simulink model "EPT"  (R2019b)
settings: Solver=FixedStepDiscrete  StartTime=0.0  StopTime=5  FixedStep=0.005  RelTol=1e-3  EnableMultiTasking=on
PreLoadFcn:
  | try, model_open; catch, disp('Error occurred while executing model pre-load callback: model_open.m'); disp('Please assure that the MATLAB working directory is set to the model directory before opening.'); end
InitFcn:
  | try, model_open; catch, end
undefined symbols (not defined in the file or in its folder): Bridge, GCM, H, ln, raptor_get_param_eval, raptor_get_safe_string, raptor_xcp_function
libraries: Raptor_lib x2810, simulink x374, hdlsllib x19
(part 16 of 45)

== system EPT/Foreground_TimeBase_5ms/CAN/CAN2_exec/BCU vs ITRI//ARTC/Remote DAG2-5EA ==
  Enable : EnablePort
  Trigger : TriggerPort  VariantControl=Variant  PortDimensions=1
  Data Type Conversion{1..8} (8 alike) : DataTypeConversion
  Fcn{1..8} (8 alike) : Fcn  Expr=(u(1)+40)/0.5
  raptor_can_txmsg : Raptor_lib/CAN/raptor_can_txmsg  canDefinition=struct('dbcFile', 'BCUvsRMDA_CMU.dbc','message', 'RemoteDAG_5EA','comment', '','signals', {{'CMU2_Tcell_T01','CMU2_Tcell_T02','CMU2_Tcell_T03','CMU2_Tcell_T04','CMU2_Tcell_T05','CMU2_Tcell_T06','CMU2_Tcell_T07','CMU2_Tcell_T08'}},'enabled', [ 1 1 1 1 1 1 1 1;],'canBus', '''CAN2''','messageID', [ 1514;],'idMask', [ 536870911;],'payloadMask', [],'payloadValue', [],'period', [ 0;],'mailbox', '','queueSize', [ 1;],'label', [ 0;],'ver', [ 2;],'showID', [ 0;],'showRaw', [ 0;],'fill', [ 0;],'editID', [ 0;],'signalOrder', [ 1;])  canBus='CAN2'  queueSize=1  payloadMask=[]  payloadValue=[]  period=0  showID=0  label=0  idMask=hex2dec('1FFFFFFF')  fill=0  id=1514  showRaw=0  signalOrder=1  signalInfo={{struct('Name', 'CMU2_Tcell_T01','Startbit', [ 0;],'SignalSize', [ 8;],'ByteOrder', 'BigEndian','ValueType', 'UNSIGNED','Class', 'uint8','Signed', [ 0;],'Factor', [ 1;],'Offset', [ 0;],'Min', [ 0;],'Max', [ 0;],'Units', '','Comment', '','StartBit', [ 0;]),struct('Name', 'CMU2_Tcell_T02','Startbit', [ 0;],'SignalSize', [ 8;],'ByteOrder', 'BigEndian','ValueType', 'UNSIGNED','Class', 'uint8','Signed', [ 0;],'Factor', [ 1;],'Offset', [ 0;],'Min', [ 0;],'Max', [ 0;],'Units', '','Comment', '','StartBit', [ 8;]),struct('Name', 'CMU2_Tcell_T03','Startbit', [ 0;],'SignalSize', [ 8;],'ByteOrder', 'BigEndian','ValueType', 'UNSIGNED','Class', 'uint8','Signed', [ 0;],'Factor', [ 1;],'Offset', [ 0;],'Min', [ 0;],'Max', [ 0;],'Units', '','Comment', '','StartBit', [ 16;]),struct('Name', 'CMU2_Tcell_T04','Startbit', [ 0;],'SignalSize', [ 8;],'ByteOrder', 'BigEndian','ValueType', 'UNSIGNED','Class', 'uint8','Signed', [ 0;],'Factor', [ 1;],'Offset', [ 0;],'Min', [ 0;],'Max', [ 0;],'Units', '','Comment', '','StartBit', [ 24;]),struct('Name', 'CMU2_Tcell_T05','Startbit', [ 0;],'SignalSize', [ 8;],'ByteOrder', 'BigEndian','ValueType', 'UNSIGNED','Class', 'uint8','Signed', [ 0;],'Factor', [ 1;],'Offset', [ 0;],'Min', [ 0;],'Max', [ 0;],'Units', '','Comment', '','StartBit', [ 32;]),struct('Name', 'CMU2_Tcell_T06','Startbit', [ 0;],'SignalSize', [ 8;],'ByteOrder', 'BigEndian','ValueType', 'UNSIGNED','Class', 'uint8','Signed', [ 0;],'Factor', [ 1;],'Offset', [ 0;],'Min', [ 0;],'Max', [ 0;],'Units', '','Comment', '','StartBit', [ 40;]),struct('Name', 'CMU2_Tcell_T07','Startbit', [ 0;],'SignalSize', [ 8;],'ByteOrder', 'BigEndian','ValueType', 'UNSIGNED','Class', 'uint8','Signed', [ 0;],'Factor', [ 1;],'Offset', [ 0;],'Min', [ 0;],'Max', [ 0;],'Units', '','Comment', '','StartBit', [ 48;]),struct('Name', 'CMU2_Tcell_T08','Startbit', [ 0;],'SignalSize', [ 8;],'ByteOrder', 'BigEndian','ValueType', 'UNSIGNED','Class', 'uint8','Signed', [ 0;],'Factor', [ 1;],'Offset', [ 0;],'Min', [ 0;],'Max', [ 0;],'Units', '','Comment', '','StartBit', [ 56;])}}
      settings: SourceProductName=Raptor
  raptor_data_read1 : Raptor_lib/Data Storage/raptor_data_read  dataName='CMU2_CELL02_TEMP'  dataShape=Scalar  idxSource=Input  idxRow=1  idxCol=1
      settings: SourceProductName=Raptor
  raptor_data_read2 : Raptor_lib/Data Storage/raptor_data_read  dataName='CMU2_CELL03_TEMP'  dataShape=Scalar  idxSource=Input  idxRow=1  idxCol=1
      settings: SourceProductName=Raptor
  raptor_data_read3 : Raptor_lib/Data Storage/raptor_data_read  dataName='CMU2_CELL01_TEMP'  dataShape=Scalar  idxSource=Input  idxRow=1  idxCol=1
      settings: SourceProductName=Raptor
  raptor_data_read4 : Raptor_lib/Data Storage/raptor_data_read  dataName='CMU2_CELL04_TEMP'  dataShape=Scalar  idxSource=Input  idxRow=1  idxCol=1
      settings: SourceProductName=Raptor
  raptor_data_read5 : Raptor_lib/Data Storage/raptor_data_read  dataName='CMU2_CELL05_TEMP'  dataShape=Scalar  idxSource=Input  idxRow=1  idxCol=1
      settings: SourceProductName=Raptor
  raptor_data_read6 : Raptor_lib/Data Storage/raptor_data_read  dataName='CMU2_CELL06_TEMP'  dataShape=Scalar  idxSource=Input  idxRow=1  idxCol=1
      settings: SourceProductName=Raptor
  raptor_data_read7 : Raptor_lib/Data Storage/raptor_data_read  dataName='CMU2_CELL07_TEMP'  dataShape=Scalar  idxSource=Input  idxRow=1  idxCol=1
      settings: SourceProductName=Raptor
  raptor_data_read8 : Raptor_lib/Data Storage/raptor_data_read  dataName='CMU2_CELL08_TEMP'  dataShape=Scalar  idxSource=Input  idxRow=1  idxCol=1
      settings: SourceProductName=Raptor
  wires:
  raptor_data_read4/1 -> Fcn4/1
  raptor_data_read3/1 -> Fcn2/1
  raptor_data_read6/1 -> Fcn6/1
  raptor_data_read2/1 -> Fcn3/1
  raptor_data_read5/1 -> Fcn5/1
  Data Type Conversion8/1 -> raptor_can_txmsg/8
  Fcn5/1 -> Data Type Conversion5/1
  Data Type Conversion3/1 -> raptor_can_txmsg/1
  Data Type Conversion2/1 -> raptor_can_txmsg/3
  Fcn2/1 -> Data Type Conversion3/1
  raptor_data_read7/1 -> Fcn7/1
  Data Type Conversion6/1 -> raptor_can_txmsg/6
  raptor_data_read1/1 -> Fcn1/1
  Fcn7/1 -> Data Type Conversion7/1
  Fcn6/1 -> Data Type Conversion6/1
  Fcn3/1 -> Data Type Conversion2/1
  Data Type Conversion7/1 -> raptor_can_txmsg/7
  Data Type Conversion4/1 -> raptor_can_txmsg/4
  Data Type Conversion1/1 -> raptor_can_txmsg/2
  Fcn8/1 -> Data Type Conversion8/1
  Fcn1/1 -> Data Type Conversion1/1
  Fcn4/1 -> Data Type Conversion4/1
  Data Type Conversion5/1 -> raptor_can_txmsg/5
  raptor_data_read8/1 -> Fcn8/1

== system EPT/Foreground_TimeBase_5ms/CAN/CAN2_exec/BCU vs ITRI//ARTC/Remote DAG2-5EB ==
  Enable : EnablePort
  Trigger : TriggerPort  VariantControl=Variant  PortDimensions=1
  Data Type Conversion{1..8} (8 alike) : DataTypeConversion
  Fcn{1..8} (8 alike) : Fcn  Expr=(u(1)+40)/0.5
  raptor_can_txmsg : Raptor_lib/CAN/raptor_can_txmsg  canDefinition=struct('dbcFile', 'BCUvsRMDA_CMU.dbc','message', 'RemoteDAG_5EB','comment', '','signals', {{'CMU2_Tcell_T09','CMU2_Tcell_T10','CMU2_Tcell_T11','CMU2_Tcell_T12','CMU2_Tcell_T13','CMU2_Tcell_T14','CMU2_Tcell_T15','CMU2_Tcell_T16'}},'enabled', [ 1 1 1 1 1 1 1 1;],'canBus', '''CAN2''','messageID', [ 1515;],'idMask', [ 536870911;],'payloadMask', [],'payloadValue', [],'period', [ 0;],'mailbox', '','queueSize', [ 1;],'label', [ 0;],'ver', [ 2;],'showID', [ 0;],'showRaw', [ 0;],'fill', [ 0;],'editID', [ 0;],'signalOrder', [ 1;])  canBus='CAN2'  queueSize=1  payloadMask=[]  payloadValue=[]  period=0  showID=0  label=0  idMask=hex2dec('1FFFFFFF')  fill=0  id=1515  showRaw=0  signalOrder=1  signalInfo={{struct('Name', 'CMU2_Tcell_T09','Startbit', [ 0;],'SignalSize', [ 8;],'ByteOrder', 'BigEndian','ValueType', 'UNSIGNED','Class', 'uint8','Signed', [ 0;],'Factor', [ 1;],'Offset', [ 0;],'Min', [ 0;],'Max', [ 0;],'Units', '','Comment', '','StartBit', [ 0;]),struct('Name', 'CMU2_Tcell_T10','Startbit', [ 0;],'SignalSize', [ 8;],'ByteOrder', 'BigEndian','ValueType', 'UNSIGNED','Class', 'uint8','Signed', [ 0;],'Factor', [ 1;],'Offset', [ 0;],'Min', [ 0;],'Max', [ 0;],'Units', '','Comment', '','StartBit', [ 8;]),struct('Name', 'CMU2_Tcell_T11','Startbit', [ 0;],'SignalSize', [ 8;],'ByteOrder', 'BigEndian','ValueType', 'UNSIGNED','Class', 'uint8','Signed', [ 0;],'Factor', [ 1;],'Offset', [ 0;],'Min', [ 0;],'Max', [ 0;],'Units', '','Comment', '','StartBit', [ 16;]),struct('Name', 'CMU2_Tcell_T12','Startbit', [ 0;],'SignalSize', [ 8;],'ByteOrder', 'BigEndian','ValueType', 'UNSIGNED','Class', 'uint8','Signed', [ 0;],'Factor', [ 1;],'Offset', [ 0;],'Min', [ 0;],'Max', [ 0;],'Units', '','Comment', '','StartBit', [ 24;]),struct('Name', 'CMU2_Tcell_T13','Startbit', [ 0;],'SignalSize', [ 8;],'ByteOrder', 'BigEndian','ValueType', 'UNSIGNED','Class', 'uint8','Signed', [ 0;],'Factor', [ 1;],'Offset', [ 0;],'Min', [ 0;],'Max', [ 0;],'Units', '','Comment', '','StartBit', [ 32;]),struct('Name', 'CMU2_Tcell_T14','Startbit', [ 0;],'SignalSize', [ 8;],'ByteOrder', 'BigEndian','ValueType', 'UNSIGNED','Class', 'uint8','Signed', [ 0;],'Factor', [ 1;],'Offset', [ 0;],'Min', [ 0;],'Max', [ 0;],'Units', '','Comment', '','StartBit', [ 40;]),struct('Name', 'CMU2_Tcell_T15','Startbit', [ 0;],'SignalSize', [ 8;],'ByteOrder', 'BigEndian','ValueType', 'UNSIGNED','Class', 'uint8','Signed', [ 0;],'Factor', [ 1;],'Offset', [ 0;],'Min', [ 0;],'Max', [ 0;],'Units', '','Comment', '','StartBit', [ 48;]),struct('Name', 'CMU2_Tcell_T16','Startbit', [ 0;],'SignalSize', [ 8;],'ByteOrder', 'BigEndian','ValueType', 'UNSIGNED','Class', 'uint8','Signed', [ 0;],'Factor', [ 1;],'Offset', [ 0;],'Min', [ 0;],'Max', [ 0;],'Units', '','Comment', '','StartBit', [ 56;])}}
      settings: SourceProductName=Raptor
  raptor_data_read1 : Raptor_lib/Data Storage/raptor_data_read  dataName='CMU2_CELL11_TEMP'  dataShape=Scalar  idxSource=Input  idxRow=1  idxCol=1
      settings: SourceProductName=Raptor
  raptor_data_read2 : Raptor_lib/Data Storage/raptor_data_read  dataName='CMU2_CELL09_TEMP'  dataShape=Scalar  idxSource=Input  idxRow=1  idxCol=1
      settings: SourceProductName=Raptor
  raptor_data_read3 : Raptor_lib/Data Storage/raptor_data_read  dataName='CMU2_CELL10_TEMP'  dataShape=Scalar  idxSource=Input  idxRow=1  idxCol=1
      settings: SourceProductName=Raptor
  raptor_data_read4 : Raptor_lib/Data Storage/raptor_data_read  dataName='CMU2_CELL13_TEMP'  dataShape=Scalar  idxSource=Input  idxRow=1  idxCol=1
      settings: SourceProductName=Raptor
  raptor_data_read5 : Raptor_lib/Data Storage/raptor_data_read  dataName='CMU2_CELL12_TEMP'  dataShape=Scalar  idxSource=Input  idxRow=1  idxCol=1
      settings: SourceProductName=Raptor
  raptor_data_read6 : Raptor_lib/Data Storage/raptor_data_read  dataName='CMU2_CELL15_TEMP'  dataShape=Scalar  idxSource=Input  idxRow=1  idxCol=1
      settings: SourceProductName=Raptor
  raptor_data_read7 : Raptor_lib/Data Storage/raptor_data_read  dataName='CMU2_CELL14_TEMP'  dataShape=Scalar  idxSource=Input  idxRow=1  idxCol=1
      settings: SourceProductName=Raptor
  raptor_data_read9 : Raptor_lib/Data Storage/raptor_data_read  dataName='CMU2_CELL16_TEMP'  dataShape=Scalar  idxSource=Input  idxRow=1  idxCol=1
      settings: SourceProductName=Raptor
  wires:
  raptor_data_read5/1 -> Fcn4/1
  raptor_data_read2/1 -> Fcn2/1
  raptor_data_read7/1 -> Fcn6/1
  raptor_data_read1/1 -> Fcn3/1
  raptor_data_read4/1 -> Fcn5/1
  Data Type Conversion8/1 -> raptor_can_txmsg/8
  Fcn5/1 -> Data Type Conversion5/1
  Data Type Conversion3/1 -> raptor_can_txmsg/1
  Data Type Conversion2/1 -> raptor_can_txmsg/3
  Fcn2/1 -> Data Type Conversion3/1
  raptor_data_read6/1 -> Fcn7/1
  Data Type Conversion6/1 -> raptor_can_txmsg/6
  raptor_data_read3/1 -> Fcn1/1
  Fcn7/1 -> Data Type Conversion7/1
  Fcn6/1 -> Data Type Conversion6/1
  Fcn3/1 -> Data Type Conversion2/1
  Data Type Conversion7/1 -> raptor_can_txmsg/7
  Data Type Conversion4/1 -> raptor_can_txmsg/4
  Data Type Conversion1/1 -> raptor_can_txmsg/2
  Fcn8/1 -> Data Type Conversion8/1
  Fcn1/1 -> Data Type Conversion1/1
  Fcn4/1 -> Data Type Conversion4/1
  Data Type Conversion5/1 -> raptor_can_txmsg/5
  raptor_data_read9/1 -> Fcn8/1

== system EPT/Foreground_TimeBase_5ms/CAN/CAN2_exec/ECHS/CountTrigger ==
  Counter : Inport
  Constant1 : Constant  Value=0
  Constant3 : Constant
  CycleTrigger : Subsystem
  Switch : Switch  Threshold=1
  Unit Delay1 : UnitDelay  SampleTime=-1  HasFrameUpgradeWarning=on
  Unit Delay2 : UnitDelay  SampleTime=-1  HasFrameUpgradeWarning=on
  Tirgger : Outport  VectorParamsAs1DForOutWhenUnconnected=off
  wires:
  Switch/1 -> Unit Delay1/1
  Constant3/1 -> Switch/3
  Constant1/1 -> Switch/1
  Counter/1 -> CycleTrigger/2(In2)
  CycleTrigger/1(Trigger) -> Switch/2, Unit Delay2/1
  Unit Delay1/1 -> CycleTrigger/1(In1)
  Unit Delay2/1 -> Tirgger/1

== system EPT/Foreground_TimeBase_5ms/CAN/CAN2_exec/ECHS/EPT2ECHS_RX ==
  Trigger : TriggerPort  VariantControl=Variant  PortDimensions=1
  10ms_exec : Subsystem

== system EPT/Foreground_TimeBase_5ms/CAN/CAN2_exec/ECHS/EPT2ECHS_TX ==
  Trigger : TriggerPort  VariantControl=Variant  PortDimensions=1
  100ms_exec : Subsystem
  10ms_exec : Subsystem
  500ms_exec : Subsystem

== system EPT/Foreground_TimeBase_5ms/CAN/CAN2_exec/IVT2/Coulomb Counting Method1 ==
  Ampere input : Inport
  RC input : Inport  Port=2
  20ms : Subsystem
  Constant6 : Constant  Value=4
  CountTrigger : Subsystem
  RC Output : Outport
  wires:
  CountTrigger/1(Tirgger) -> 20ms/Trigger
  Constant6/1 -> CountTrigger/1(Counter)
  Ampere input/1 -> 20ms/1(Ampere input)
  RC input/1 -> 20ms/2(RC input)
  20ms/1(RC) -> RC Output/1

== system EPT/Foreground_TimeBase_5ms/CAN/CAN2_exec/IVT2/CountTrigger ==
  Counter : Inport
  Constant1 : Constant  Value=0
  Constant3 : Constant
  CycleTrigger : Subsystem
  Switch : Switch  Threshold=1
  Unit Delay1 : UnitDelay  SampleTime=-1  HasFrameUpgradeWarning=on
  Unit Delay2 : UnitDelay  SampleTime=-1  HasFrameUpgradeWarning=on
  Tirgger : Outport  VectorParamsAs1DForOutWhenUnconnected=off
  wires:
  Unit Delay2/1 -> Tirgger/1
  Unit Delay1/1 -> CycleTrigger/1(In1)
  CycleTrigger/1(Trigger) -> Unit Delay2/1, Switch/2
  Counter/1 -> CycleTrigger/2(In2)
  Constant1/1 -> Switch/1
  Constant3/1 -> Switch/3
  Switch/1 -> Unit Delay1/1

== system EPT/Foreground_TimeBase_5ms/CAN/CAN2_exec/IVT2/CountTrigger1 ==
  Counter : Inport
  Constant1 : Constant  Value=0
  Constant3 : Constant
  CycleTrigger : Subsystem
  Switch : Switch  Threshold=1
  Unit Delay1 : UnitDelay  SampleTime=-1  HasFrameUpgradeWarning=on
  Unit Delay2 : UnitDelay  SampleTime=-1  HasFrameUpgradeWarning=on
  Tirgger : Outport  VectorParamsAs1DForOutWhenUnconnected=off
  wires:
  Switch/1 -> Unit Delay1/1
  Constant3/1 -> Switch/3
  Constant1/1 -> Switch/1
  Counter/1 -> CycleTrigger/2(In2)
  CycleTrigger/1(Trigger) -> Switch/2, Unit Delay2/1
  Unit Delay1/1 -> CycleTrigger/1(In1)
  Unit Delay2/1 -> Tirgger/1

== system EPT/Foreground_TimeBase_5ms/CAN/CAN2_exec/IVT2/Delay2 ==
  Condition : Inport
  TimeCount : Inport  Port=2
  Constant10 : Constant
  Constant11 : Constant  Value=0
  Constant8 : Constant  Value=0
  CycleTrigger : Subsystem
  Switch2 : Switch  Threshold=1
  Switch3 : Switch  Threshold=1
  Unit Delay1 : UnitDelay  SampleTime=-1  HasFrameUpgradeWarning=on
  Unit Delay2 : UnitDelay  SampleTime=-1  HasFrameUpgradeWarning=on
  Output : Outport  VectorParamsAs1DForOutWhenUnconnected=off
  wires:
  TimeCount/1 -> CycleTrigger/2(In2)
  Condition/1 -> Switch3/2
  CycleTrigger/1(Trigger) -> Switch2/2, Unit Delay1/1
  Constant8/1 -> Switch2/1
  Constant10/1 -> Switch2/3
  Switch3/1 -> CycleTrigger/1(In1)
  Constant11/1 -> Switch3/3
  Unit Delay2/1 -> Switch3/1
  Switch2/1 -> Unit Delay2/1
  Unit Delay1/1 -> Output/1

== system EPT/Foreground_TimeBase_5ms/CAN/CAN2_exec/IVT2/Delay3 ==
  Condition : Inport
  TimeCount : Inport  Port=2
  Constant10 : Constant
  Constant11 : Constant  Value=0
  Constant8 : Constant  Value=0
  CycleTrigger : Subsystem
  Switch2 : Switch  Threshold=1
  Switch3 : Switch  Threshold=1
  Unit Delay1 : UnitDelay  SampleTime=-1  HasFrameUpgradeWarning=on
  Unit Delay2 : UnitDelay  SampleTime=-1  HasFrameUpgradeWarning=on
  Output : Outport  VectorParamsAs1DForOutWhenUnconnected=off
  wires:
  Unit Delay1/1 -> Output/1
  Switch2/1 -> Unit Delay2/1
  Unit Delay2/1 -> Switch3/1
  Constant11/1 -> Switch3/3
  Switch3/1 -> CycleTrigger/1(In1)
  Constant10/1 -> Switch2/3
  Constant8/1 -> Switch2/1
  CycleTrigger/1(Trigger) -> Unit Delay1/1, Switch2/2
  Condition/1 -> Switch3/2
  TimeCount/1 -> CycleTrigger/2(In2)

== system EPT/Foreground_TimeBase_5ms/CAN/CAN2_exec/IVT2/IVT_RX_0x521  ==
  Trigger : TriggerPort  VariantControl=Variant  PortDimensions=1
  raptor_can_rxmsg : Raptor_lib/CAN/raptor_can_rxmsg  canDefinition=struct('dbcFile', 'IVT.dbc','message', 'IVT_DATA_I','comment', '','signals', {{'I_Current','Rolling_Status','Mux_ID'}},'enabled', [ 1 1 1;],'canBus', '''CAN2''','messageID', [ 1313;],'idMask', [ 536870911;],'payloadMask', [],'payloadValue', [],'period', [ 0;],'mailbox', '''''','queueSize', [ 1;],'label', [ 0;],'ver', [ 2;],'showID', [ 0;],'showRaw', [ 0;],'fill', [ 0;],'editID', [ 0;],'signalOrder', [ 2;])  canBus='CAN2'  mailbox=''  payloadMask=[]  payloadValue=[]  idMask=hex2dec('1FFFFFFF')  queueSize=1  showID=0  label=0  fill=0  id=1313  showRaw=0  showAge=1  signalOrder=2  signalInfo={{struct('Name', 'Mux_ID','Startbit', [ 0;],'SignalSize', [ 8;],'ByteOrder', 'BigEndian','ValueType', 'UNSIGNED','Class', 'uint8','Signed', [ 0;],'Factor', [ 1;],'Offset', [ 0;],'Min', [ 0;],'Max', [ 7;],'Units', '','Comment', 'Channel NO.0~7;ID=0 for I_Current','StartBit', [ 0;]),struct('Name', 'Rolling_Status','Startbit', [ 0;],'SignalSize', [ 8;],'ByteOrder', 'BigEndian','ValueType', 'UNSIGNED','Class', 'uint8','Signed', [ 0;],'Factor', [ 1;],'Offset', [ 0;],'Min', [ 0;],'Max', [ 255;],'Units', '','Comment', 'bit0~3 RC=0~15','StartBit', [ 8;]),struct('Name', 'I_Current','Startbit', [ 0;],'SignalSize', [ 32;],'ByteOrder', 'BigEndian','ValueType', 'SIGNED','Class', 'int32','Signed', [ 1;],'Factor', [ 0.001;],'Offset', [ 0;],'Min', [ -1000;],'Max', [ 1000;],'Units', 'A','Comment', '','StartBit', [ 40;])}}
      settings: SourceProductName=Raptor
  raptor_measurement : Raptor_lib/Data Storage/raptor_measurement  paramName='PWCU_I_Current'  nameSource=Parameter  calDispType=Number  calEnum={'False', 'True'}  calGain=1.0  calOffset=0.0  calMax=inf  calMin=-inf  calFormat='-1'  calUnit=''  calHelp=''  calAccess=1  calFunction=raptor_xcp_function(gcb)  calVisible=on
      settings: SourceProductName=Raptor
  raptor_measurement1 : Raptor_lib/Data Storage/raptor_measurement  paramName='PWCU_0x521_Rolling_Status'  nameSource=Parameter  calDispType=Number  calEnum={'False', 'True'}  calGain=1.0  calOffset=0.0  calMax=inf  calMin=-inf  calFormat='-1'  calUnit=''  calHelp=''  calAccess=1  calFunction=raptor_xcp_function(gcb)  calVisible=on
      settings: SourceProductName=Raptor
  raptor_measurement2 : Raptor_lib/Data Storage/raptor_measurement  paramName='PWCU_0x521_Mux_ID'  nameSource=Parameter  calDispType=Number  calEnum={'False', 'True'}  calGain=1.0  calOffset=0.0  calMax=inf  calMin=-inf  calFormat='-1'  calUnit=''  calHelp=''  calAccess=1  calFunction=raptor_xcp_function(gcb)  calVisible=on
      settings: SourceProductName=Raptor
  raptor_measurement3 : Raptor_lib/Data Storage/raptor_measurement  paramName='PWCU_Age_0x521'  nameSource=Parameter  calDispType=Number  calEnum={'False', 'True'}  calGain=1.0  calOffset=0.0  calMax=inf  calMin=-inf  calFormat='-1'  calUnit=''  calHelp=''  calAccess=1  calFunction=raptor_xcp_function(gcb)  calVisible=on
      settings: SourceProductName=Raptor
  Current : Outport
  wires:
  raptor_can_rxmsg/4 -> raptor_measurement2/1
  raptor_can_rxmsg/1 -> raptor_measurement3/1
  raptor_can_rxmsg/3 -> raptor_measurement1/1
  raptor_can_rxmsg/2 -> Current/1, raptor_measurement/1

== system EPT/Foreground_TimeBase_5ms/CAN/CAN2_exec/IVT2/IVT_RX_0x522 ==
  Trigger : TriggerPort  TriggerType=falling  VariantControl=Variant  PortDimensions=1
  Compare To Constant : simulink/Logic and Bit Operations/Compare To Constant  relop=>=  const=1000  OutDataTypeStr=boolean
  Constant : Constant  Value=5
  Delay : Delay  DelayLength=1  InitialCondition=0
  Delay1 : Delay  DelayLength=1  InitialCondition=0
  Delay2 : Delay  InitialCondition=0
  Delay3 : Delay  DelayLength=3  InitialCondition=0
  Delay4 : Delay  DelayLength=4  InitialCondition=0
  Divide : Product  Inputs=*/
  Mux : Mux  Inputs=5
  Sum of Elements : Sum  Inputs=+
  Switch : Switch  Criteria=u2 > Threshold
  raptor_can_rxmsg1 : Raptor_lib/CAN/raptor_can_rxmsg  canDefinition=struct('dbcFile', 'IVT.dbc','message', 'IVT_DATA_U1','comment', '','signals', {{'U1_Voltage','Rolling_Status','Mux_ID'}},'enabled', [ 1 1 1;],'canBus', '''CAN2''','messageID', [ 1314;],'idMask', [ 536870911;],'payloadMask', [],'payloadValue', [],'period', [ 0;],'mailbox', '''''','queueSize', [ 1;],'label', [ 0;],'ver', [ 2;],'showID', [ 0;],'showRaw', [ 0;],'fill', [ 0;],'editID', [ 0;],'signalOrder', [ 2;])  canBus='CAN2'  mailbox=''  payloadMask=[]  payloadValue=[]  idMask=hex2dec('1FFFFFFF')  queueSize=1  showID=0  label=0  fill=0  id=1314  showRaw=0  showAge=1  signalOrder=2  signalInfo={{struct('Name', 'Mux_ID','Startbit', [ 0;],'SignalSize', [ 8;],'ByteOrder', 'BigEndian','ValueType', 'UNSIGNED','Class', 'uint8','Signed', [ 0;],'Factor', [ 1;],'Offset', [ 0;],'Min', [ 0;],'Max', [ 7;],'Units', '','Comment', 'Channel NO.0~7;ID=0 for U1','StartBit', [ 0;]),struct('Name', 'Rolling_Status','Startbit', [ 0;],'SignalSize', [ 8;],'ByteOrder', 'BigEndian','ValueType', 'UNSIGNED','Class', 'uint8','Signed', [ 0;],'Factor', [ 1;],'Offset', [ 0;],'Min', [ 0;],'Max', [ 255;],'Units', '','Comment', 'bit0~3 RC=0~15','StartBit', [ 8;]),struct('Name', 'U1_Voltage','Startbit', [ 0;],'SignalSize', [ 32;],'ByteOrder', 'BigEndian','ValueType', 'SIGNED','Class', 'int32','Signed', [ 1;],'Factor', [ 0.001;],'Offset', [ 0;],'Min', [ -1000;],'Max', [ 1000;],'Units', 'V','Comment', '','StartBit', [ 40;])}}
      settings: SourceProductName=Raptor
  raptor_measurement1 : Raptor_lib/Data Storage/raptor_measurement  paramName='PWCU_0x522_Age'  nameSource=Parameter  calDispType=Number  calEnum={'False', 'True'}  calGain=1.0  calOffset=0.0  calMax=inf  calMin=-inf  calFormat='-1'  calUnit=''  calHelp=''  calAccess=1  calFunction=raptor_xcp_function(gcb)  calVisible=on
      settings: SourceProductName=Raptor
  raptor_measurement2 : Raptor_lib/Data Storage/raptor_measurement  paramName='PWCU_U1_Voltage'  nameSource=Parameter  calDispType=Number  calEnum={'False', 'True'}  calGain=1.0  calOffset=0.0  calMax=inf  calMin=-inf  calFormat='-1'  calUnit=''  calHelp=''  calAccess=1  calFunction=raptor_xcp_function(gcb)  calVisible=on
      settings: SourceProductName=Raptor
  raptor_measurement4 : Raptor_lib/Data Storage/raptor_measurement  paramName='PWCU_0x522_Mux_ID'  nameSource=Parameter  calDispType=Number  calEnum={'False', 'True'}  calGain=1.0  calOffset=0.0  calMax=inf  calMin=-inf  calFormat='-1'  calUnit=''  calHelp=''  calAccess=1  calFunction=raptor_xcp_function(gcb)  calVisible=on
      settings: SourceProductName=Raptor
  raptor_measurement5 : Raptor_lib/Data Storage/raptor_measurement  paramName='PWCU_0x522_Rolling_Status'  nameSource=Parameter  calDispType=Number  calEnum={'False', 'True'}  calGain=1.0  calOffset=0.0  calMax=inf  calMin=-inf  calFormat='-1'  calUnit=''  calHelp=''  calAccess=1  calFunction=raptor_xcp_function(gcb)  calVisible=on
      settings: SourceProductName=Raptor
  U1_Voltage : Outport
  wires:
  Switch/1 -> Delay4/1, Delay3/1, Delay2/1, Delay1/1, Mux/1, Delay/1
  Compare To Constant/1 -> Switch/2
  raptor_can_rxmsg1/4 -> raptor_measurement4/1
  raptor_can_rxmsg1/3 -> raptor_measurement5/1
  raptor_can_rxmsg1/2 -> Compare To Constant/1, Switch/3
  raptor_can_rxmsg1/1 -> raptor_measurement1/1
  Delay/1 -> Switch/1
  Mux/1 -> Sum of Elements/1
  Delay4/1 -> Mux/5
  Delay3/1 -> Mux/4
  Delay2/1 -> Mux/3
  Delay1/1 -> Mux/2
  Sum of Elements/1 -> Divide/1
  Divide/1 -> raptor_measurement2/1, U1_Voltage/1
  Constant/1 -> Divide/2

== system EPT/Foreground_TimeBase_5ms/CAN/CAN2_exec/IVT2/IVT_RX_0x523 ==
  Trigger : TriggerPort  VariantControl=Variant  PortDimensions=1
  Compare To Constant : simulink/Logic and Bit Operations/Compare To Constant  relop=>=  const=1000  OutDataTypeStr=boolean
  Constant : Constant  Value=5
  Delay : Delay  DelayLength=1  InitialCondition=0
  Delay1 : Delay  DelayLength=1  InitialCondition=0
  Delay2 : Delay  InitialCondition=0
  Delay3 : Delay  DelayLength=3  InitialCondition=0
  Delay4 : Delay  DelayLength=4  InitialCondition=0
  Divide : Product  Inputs=*/
  Mux : Mux  Inputs=5
  Sum of Elements : Sum  Inputs=+
  Switch : Switch  Criteria=u2 > Threshold
  raptor_can_rxmsg2 : Raptor_lib/CAN/raptor_can_rxmsg  canDefinition=struct('dbcFile', 'IVT.dbc','message', 'IVT_DATA_U2','comment', '','signals', {{'U2_Voltage','Rolling_Status','Mux_ID'}},'enabled', [ 1 1 1;],'canBus', '''CAN2''','messageID', [ 1315;],'idMask', [ 536870911;],'payloadMask', [],'payloadValue', [],'period', [ 0;],'mailbox', '''''','queueSize', [ 1;],'label', [ 0;],'ver', [ 2;],'showID', [ 0;],'showRaw', [ 0;],'fill', [ 0;],'editID', [ 0;],'signalOrder', [ 2;])  canBus='CAN2'  mailbox=''  payloadMask=[]  payloadValue=[]  idMask=hex2dec('1FFFFFFF')  queueSize=1  showID=0  label=0  fill=0  id=1315  showRaw=0  showAge=1  signalOrder=2  signalInfo={{struct('Name', 'Mux_ID','Startbit', [ 0;],'SignalSize', [ 8;],'ByteOrder', 'BigEndian','ValueType', 'UNSIGNED','Class', 'uint8','Signed', [ 0;],'Factor', [ 1;],'Offset', [ 0;],'Min', [ 0;],'Max', [ 7;],'Units', '','Comment', 'Channel NO.0~7;ID=0 for U2','StartBit', [ 0;]),struct('Name', 'Rolling_Status','Startbit', [ 0;],'SignalSize', [ 8;],'ByteOrder', 'BigEndian','ValueType', 'UNSIGNED','Class', 'uint8','Signed', [ 0;],'Factor', [ 1;],'Offset', [ 0;],'Min', [ 0;],'Max', [ 255;],'Units', '','Comment', 'bit0~3 RC=0~15','StartBit', [ 8;]),struct('Name', 'U2_Voltage','Startbit', [ 0;],'SignalSize', [ 32;],'ByteOrder', 'BigEndian','ValueType', 'SIGNED','Class', 'int32','Signed', [ 1;],'Factor', [ 0.001;],'Offset', [ 0;],'Min', [ -1000;],'Max', [ 1000;],'Units', 'V','Comment', '','StartBit', [ 40;])}}
      settings: SourceProductName=Raptor
  raptor_measurement1 : Raptor_lib/Data Storage/raptor_measurement  paramName='PWCU_0x523_Age'  nameSource=Parameter  calDispType=Number  calEnum={'False', 'True'}  calGain=1.0  calOffset=0.0  calMax=inf  calMin=-inf  calFormat='-1'  calUnit=''  calHelp=''  calAccess=1  calFunction=raptor_xcp_function(gcb)  calVisible=on
      settings: SourceProductName=Raptor
  raptor_measurement2 : Raptor_lib/Data Storage/raptor_measurement  paramName='PWCU_U2_Voltage'  nameSource=Parameter  calDispType=Number  calEnum={'False', 'True'}  calGain=1.0  calOffset=0.0  calMax=inf  calMin=-inf  calFormat='-1'  calUnit=''  calHelp=''  calAccess=1  calFunction=raptor_xcp_function(gcb)  calVisible=on
      settings: SourceProductName=Raptor
  raptor_measurement4 : Raptor_lib/Data Storage/raptor_measurement  paramName='PWCU_0x523_Mux_ID'  nameSource=Parameter  calDispType=Number  calEnum={'False', 'True'}  calGain=1.0  calOffset=0.0  calMax=inf  calMin=-inf  calFormat='-1'  calUnit=''  calHelp=''  calAccess=1  calFunction=raptor_xcp_function(gcb)  calVisible=on
      settings: SourceProductName=Raptor
  raptor_measurement5 : Raptor_lib/Data Storage/raptor_measurement  paramName='PWCU_0x523_Rolling_Status'  nameSource=Parameter  calDispType=Number  calEnum={'False', 'True'}  calGain=1.0  calOffset=0.0  calMax=inf  calMin=-inf  calFormat='-1'  calUnit=''  calHelp=''  calAccess=1  calFunction=raptor_xcp_function(gcb)  calVisible=on
      settings: SourceProductName=Raptor
  wires:
  Compare To Constant/1 -> Switch/2
  raptor_can_rxmsg2/2 -> Switch/3, Compare To Constant/1
  raptor_can_rxmsg2/4 -> raptor_measurement4/1
  raptor_can_rxmsg2/1 -> raptor_measurement1/1
  raptor_can_rxmsg2/3 -> raptor_measurement5/1
  Delay/1 -> Switch/1
  Delay2/1 -> Mux/3
  Delay3/1 -> Mux/4
  Switch/1 -> Mux/1, Delay1/1, Delay2/1, Delay4/1, Delay3/1, Delay/1
  Delay1/1 -> Mux/2
  Sum of Elements/1 -> Divide/1
  Mux/1 -> Sum of Elements/1
  Delay4/1 -> Mux/5
  Divide/1 -> raptor_measurement2/1
  Constant/1 -> Divide/2

== system EPT/Foreground_TimeBase_5ms/CAN/CAN2_exec/IVT2/IVT_RX_0x524 ==
  Trigger : TriggerPort  TriggerType=falling  VariantControl=Variant  PortDimensions=1
  Compare To Constant : simulink/Logic and Bit Operations/Compare To Constant  relop=>=  const=1000  OutDataTypeStr=boolean
  Constant : Constant  Value=5
  Delay : Delay  DelayLength=1  InitialCondition=0
  Delay1 : Delay  DelayLength=1  InitialCondition=0
  Delay2 : Delay  InitialCondition=0
  Delay3 : Delay  DelayLength=3  InitialCondition=0
  Delay4 : Delay  DelayLength=4  InitialCondition=0
  Divide : Product  Inputs=*/
  Mux : Mux  Inputs=5
  Sum of Elements : Sum  Inputs=+
  Switch : Switch  Criteria=u2 > Threshold
  raptor_can_rxmsg3 : Raptor_lib/CAN/raptor_can_rxmsg  canDefinition=struct('dbcFile', 'IVT.dbc','message', 'IVT_DATA_U3','comment', '','signals', {{'U3_Voltage','Rolling_Status','Mux_ID'}},'enabled', [ 1 1 1;],'canBus', '''CAN2''','messageID', [ 1316;],'idMask', [ 536870911;],'payloadMask', [],'payloadValue', [],'period', [ 0;],'mailbox', '''''','queueSize', [ 1;],'label', [ 0;],'ver', [ 2;],'showID', [ 0;],'showRaw', [ 0;],'fill', [ 0;],'editID', [ 0;],'signalOrder', [ 2;])  canBus='CAN2'  mailbox=''  payloadMask=[]  payloadValue=[]  idMask=hex2dec('1FFFFFFF')  queueSize=1  showID=0  label=0  fill=0  id=1316  showRaw=0  showAge=1  signalOrder=2  signalInfo={{struct('Name', 'Mux_ID','Startbit', [ 0;],'SignalSize', [ 8;],'ByteOrder', 'BigEndian','ValueType', 'UNSIGNED','Class', 'uint8','Signed', [ 0;],'Factor', [ 1;],'Offset', [ 0;],'Min', [ 0;],'Max', [ 0;],'Units', '','Comment', 'Channel NO.0~7;ID=0 for U3','StartBit', [ 0;]),struct('Name', 'Rolling_Status','Startbit', [ 0;],'SignalSize', [ 8;],'ByteOrder', 'BigEndian','ValueType', 'UNSIGNED','Class', 'uint8','Signed', [ 0;],'Factor', [ 1;],'Offset', [ 0;],'Min', [ 0;],'Max', [ 255;],'Units', '','Comment', 'bit0~3 RC=0~15','StartBit', [ 8;]),struct('Name', 'U3_Voltage','Startbit', [ 0;],'SignalSize', [ 32;],'ByteOrder', 'BigEndian','ValueType', 'SIGNED','Class', 'int32','Signed', [ 1;],'Factor', [ 0.001;],'Offset', [ 0;],'Min', [ -1000;],'Max', [ 1000;],'Units', 'V','Comment', '','StartBit', [ 40;])}}
      settings: SourceProductName=Raptor
  raptor_measurement1 : Raptor_lib/Data Storage/raptor_measurement  paramName='PWCU_0x524_Age'  nameSource=Parameter  calDispType=Number  calEnum={'False', 'True'}  calGain=1.0  calOffset=0.0  calMax=inf  calMin=-inf  calFormat='-1'  calUnit=''  calHelp=''  calAccess=1  calFunction=raptor_xcp_function(gcb)  calVisible=on
      settings: SourceProductName=Raptor
  raptor_measurement2 : Raptor_lib/Data Storage/raptor_measurement  paramName='PWCU_U3_Voltage'  nameSource=Parameter  calDispType=Number  calEnum={'False', 'True'}  calGain=1.0  calOffset=0.0  calMax=inf  calMin=-inf  calFormat='-1'  calUnit=''  calHelp=''  calAccess=1  calFunction=raptor_xcp_function(gcb)  calVisible=on
      settings: SourceProductName=Raptor
  raptor_measurement4 : Raptor_lib/Data Storage/raptor_measurement  paramName='PWCU_0x524_Mux_ID'  nameSource=Parameter  calDispType=Number  calEnum={'False', 'True'}  calGain=1.0  calOffset=0.0  calMax=inf  calMin=-inf  calFormat='-1'  calUnit=''  calHelp=''  calAccess=1  calFunction=raptor_xcp_function(gcb)  calVisible=on
      settings: SourceProductName=Raptor
  raptor_measurement5 : Raptor_lib/Data Storage/raptor_measurement  paramName='PWCU_0x524_Rolling_Status'  nameSource=Parameter  calDispType=Number  calEnum={'False', 'True'}  calGain=1.0  calOffset=0.0  calMax=inf  calMin=-inf  calFormat='-1'  calUnit=''  calHelp=''  calAccess=1  calFunction=raptor_xcp_function(gcb)  calVisible=on
      settings: SourceProductName=Raptor
  wires:
  Compare To Constant/1 -> Switch/2
  raptor_can_rxmsg3/2 -> Compare To Constant/1, Switch/3
  raptor_can_rxmsg3/1 -> raptor_measurement1/1
  raptor_can_rxmsg3/4 -> raptor_measurement4/1
  raptor_can_rxmsg3/3 -> raptor_measurement5/1
  Delay/1 -> Switch/1
  Switch/1 -> Mux/1, Delay4/1, Delay3/1, Delay2/1, Delay1/1, Delay/1
  Divide/1 -> raptor_measurement2/1
  Mux/1 -> Sum of Elements/1
  Delay4/1 -> Mux/5
  Delay1/1 -> Mux/2
  Constant/1 -> Divide/2
  Sum of Elements/1 -> Divide/1
  Delay2/1 -> Mux/3
  Delay3/1 -> Mux/4

== system EPT/Foreground_TimeBase_5ms/CAN/CAN2_exec/IVT2/Latch ==
  Latch : Inport
  Reset : Inport  Port=2
  Switch1 : Switch  Criteria=u2 > Threshold
  Switch3 : Switch  Criteria=u2 > Threshold
  Unit Delay1 : UnitDelay  SampleTime=-1  HasFrameUpgradeWarning=on
  Output : Outport  VectorParamsAs1DForOutWhenUnconnected=off
  wires:
  Unit Delay1/1 -> Switch1/3
  Switch3/1 -> Output/1, Unit Delay1/1
  Reset/1 -> Switch3/2
  Latch/1 -> Switch1/1, Switch1/2
  Switch1/1 -> Switch3/3

== system EPT/Foreground_TimeBase_5ms/CAN/CAN2_exec/IVT2/Latch1 ==
  Latch : Inport
  Reset : Inport  Port=2
  Switch1 : Switch  Criteria=u2 > Threshold
  Switch3 : Switch  Criteria=u2 > Threshold
  Unit Delay1 : UnitDelay  SampleTime=-1  HasFrameUpgradeWarning=on
  Output : Outport  VectorParamsAs1DForOutWhenUnconnected=off
  wires:
  Switch1/1 -> Switch3/3
  Latch/1 -> Switch1/2, Switch1/1
  Reset/1 -> Switch3/2
  Switch3/1 -> Unit Delay1/1, Output/1
  Unit Delay1/1 -> Switch1/3

== system EPT/Foreground_TimeBase_5ms/CAN/CAN2_exec/Remote DA /CountTrigger ==
  Counter : Inport
  Constant1 : Constant  Value=0
  Constant3 : Constant
  CycleTrigger : Subsystem
  Switch : Switch  Threshold=1
  Unit Delay1 : UnitDelay  SampleTime=-1  HasFrameUpgradeWarning=on
  Unit Delay2 : UnitDelay  SampleTime=-1  HasFrameUpgradeWarning=on
  Tirgger : Outport  VectorParamsAs1DForOutWhenUnconnected=off
  wires:
  Unit Delay2/1 -> Tirgger/1
  Unit Delay1/1 -> CycleTrigger/1(In1)
  CycleTrigger/1(Trigger) -> Unit Delay2/1, Switch/2
  Counter/1 -> CycleTrigger/2(In2)
  Constant1/1 -> Switch/1
  Constant3/1 -> Switch/3
  Switch/1 -> Unit Delay1/1

== system EPT/Foreground_TimeBase_5ms/CAN/CAN2_exec/Remote DA /Remote DA Status G13 (Vehicle-EPT_OP_Status#1) ==
  Trigger : TriggerPort  VariantControl=Variant  PortDimensions=1
  raptor_can_txmsg : Raptor_lib/CAN/raptor_can_txmsg  canDefinition=struct('dbcFile', 'EPTvsRemoteDA.dbc','message', 'Remote_DA_Status_G13','comment', '','signals', {{'EPT_VEH_MODE_STA_DUP','EPT_GEAR_STA_DUP','EPT_TRQ_CMD_DUP','EPT_MOTOR_SPD_DUP','EPT_MCU_DC_VOLT','EPT_MCU_RMS_CURR'}},'enabled', [ 1 1 1 1 1 1;],'canBus', '''CAN2''','messageID', [ 403959540;],'idMask', [ 536870911;],'payloadMask', [],'payloadValue', [],'period', [ 0;],'mailbox', '','queueSize', [ 1;],'label', [ 0;],'ver', [ 2;],'showID', [ 0;],'showRaw', [ 0;],'fill', [ 0;],'editID', [ 0;],'signalOrder', [ 2;])  canBus='CAN2'  queueSize=1  payloadMask=[]  payloadValue=[]  period=0  showID=0  label=0  idMask=hex2dec('1FFFFFFF')  fill=0  id=403959540  showRaw=0  signalOrder=2  signalInfo={{struct('Name', 'EPT_MCU_RMS_CURR','Startbit', [ 0;],'SignalSize', [ 16;],'ByteOrder', 'LittleEndian','ValueType', 'UNSIGNED','Class', 'uint16','Signed', [ 0;],'Factor', [ 1;],'Offset', [ -1000;],'Min', [ -1000;],'Max', [ 1000;],'Units', 'A','Comment', '','StartBit', [ 40;]),struct('Name', 'EPT_MCU_DC_VOLT','Startbit', [ 0;],'SignalSize', [ 8;],'ByteOrder', 'LittleEndian','ValueType', 'UNSIGNED','Class', 'uint8','Signed', [ 0;],'Factor', [ 0.4;],'Offset', [ 0;],'Min', [ 0;],'Max', [ 100;],'Units', '%(Max_Vbatt)','Comment', '','StartBit', [ 32;]),struct('Name', 'EPT_MOTOR_SPD_DUP','Startbit', [ 0;],'SignalSize', [ 16;],'ByteOrder', 'LittleEndian','ValueType', 'UNSIGNED','Class', 'uint16','Signed', [ 0;],'Factor', [ 1;],'Offset', [ -12000;],'Min', [ -12000;],'Max', [ 12000;],'Units', 'rpm','Comment', '','StartBit', [ 16;]),struct('Name', 'EPT_TRQ_CMD_DUP','Startbit', [ 0;],'SignalSize', [ 8;],'ByteOrder', 'LittleEndian','ValueType', 'UNSIGNED','Class', 'uint8','Signed', [ 0;],'Factor', [ 0.4;],'Offset', [ 0;],'Min', [ 0;],'Max', [ 100;],'Units', 'pct','Comment', '','StartBit', [ 8;]),struct('Name', 'EPT_GEAR_STA_DUP','Startbit', [ 0;],'SignalSize', [ 4;],'ByteOrder', 'LittleEndian','ValueType', 'UNSIGNED','Class', 'uint8','Signed', [ 0;],'Factor', [ 1;],'Offset', [ 0;],'Min', [ 0;],'Max', [ 0;],'Units', '','Comment', '','StartBit', [ 4;]),struct('Name', 'EPT_VEH_MODE_STA_DUP','Startbit', [ 0;],'SignalSize', [ 2;],'ByteOrder', 'LittleEndian','ValueType', 'UNSIGNED','Class', 'uint8','Signed', [ 0;],'Factor', [ 1;],'Offset', [ 0;],'Min', [ 0;],'Max', [ 0;],'Units', '','Comment', '','StartBit', [ 0;])}}
      settings: SourceProductName=Raptor
  raptor_data_read1 : Raptor_lib/Data Storage/raptor_data_read  dataName='Read_AC_Motor_Current'  dataShape=Scalar  idxSource=Input  idxRow=1  idxCol=1
      settings: SourceProductName=Raptor
  raptor_data_read2 : Raptor_lib/Data Storage/raptor_data_read  dataName='EPT_MOTOR_SPD'  dataShape=Scalar  idxSource=Input  idxRow=1  idxCol=1
      settings: SourceProductName=Raptor
  raptor_data_read3 : Raptor_lib/Data Storage/raptor_data_read  dataName='ECHS_TRQ_CMD'  dataShape=Scalar  idxSource=Input  idxRow=1  idxCol=1
      settings: SourceProductName=Raptor
  raptor_data_read5 : Raptor_lib/Data Storage/raptor_data_read  dataName='EPT_GEAR_STA'  dataShape=Scalar  idxSource=Input  idxRow=1  idxCol=1
      settings: SourceProductName=Raptor
  raptor_data_read7 : Raptor_lib/Data Storage/raptor_data_read  dataName='EPT_VEH_MODE_STA'  dataShape=Scalar  idxSource=Input  idxRow=1  idxCol=1
      settings: SourceProductName=Raptor
  raptor_data_read9 : Raptor_lib/Data Storage/raptor_data_read  dataName='Read_Controller_Cap_Voltage'  dataShape=Scalar  idxSource=Input  idxRow=1  idxCol=1
      settings: SourceProductName=Raptor
  wires:
  raptor_data_read1/1 -> raptor_can_txmsg/6
  raptor_data_read9/1 -> raptor_can_txmsg/5
  raptor_data_read2/1 -> raptor_can_txmsg/4
  raptor_data_read3/1 -> raptor_can_txmsg/3
  raptor_data_read5/1 -> raptor_can_txmsg/2
  raptor_data_read7/1 -> raptor_can_txmsg/1

== system EPT/Foreground_TimeBase_5ms/CAN/CAN2_exec/Remote DA /Remote DA Status G14 (Vehicle-EPT_OP_Status#2) ==
  Trigger : TriggerPort  VariantControl=Variant  PortDimensions=1
  raptor_can_txmsg : Raptor_lib/CAN/raptor_can_txmsg  canDefinition=struct('dbcFile', 'EPTvsRemoteDA.dbc','message', 'Remote_DA_Status_G14','comment', '','signals', {{'EPT_MOTOR_TEMP_DUP','EPT_MCU_TEMP_DUP','EPT_MCU_FAULT_LEVEL','EPT_MCU_FAULT_CAUSE','EPT_MCU_FAULT_ID'}},'enabled', [ 1 1 1 1 1;],'canBus', '''CAN2''','messageID', [ 404029428;],'idMask', [ 536870911;],'payloadMask', [],'payloadValue', [],'period', [ 0;],'mailbox', '','queueSize', [ 1;],'label', [ 1;],'ver', [ 2;],'showID', [ 0;],'showRaw', [ 0;],'fill', [ 0;],'editID', [ 0;],'signalOrder', [ 2;])  canBus='CAN2'  queueSize=1  payloadMask=[]  payloadValue=[]  period=0  showID=0  label=1  idMask=hex2dec('1FFFFFFF')  fill=0  id=404029428  showRaw=0  signalOrder=2  signalInfo={{struct('Name', 'EPT_MCU_FAULT_ID','Startbit', [ 0;],'SignalSize', [ 16;],'ByteOrder', 'LittleEndian','ValueType', 'UNSIGNED','Class', 'uint16','Signed', [ 0;],'Factor', [ 1;],'Offset', [ 0;],'Min', [ 0;],'Max', [ 0;],'Units', '','Comment', '','StartBit', [ 48;]),struct('Name', 'EPT_MCU_FAULT_CAUSE','Startbit', [ 0;],'SignalSize', [ 8;],'ByteOrder', 'LittleEndian','ValueType', 'UNSIGNED','Class', 'uint8','Signed', [ 0;],'Factor', [ 1;],'Offset', [ 0;],'Min', [ 0;],'Max', [ 0;],'Units', '','Comment', '','StartBit', [ 40;]),struct('Name', 'EPT_MCU_FAULT_LEVEL','Startbit', [ 0;],'SignalSize', [ 4;],'ByteOrder', 'LittleEndian','ValueType', 'UNSIGNED','Class', 'uint8','Signed', [ 0;],'Factor', [ 1;],'Offset', [ 0;],'Min', [ 0;],'Max', [ 0;],'Units', '','Comment', '','StartBit', [ 32;]),struct('Name', 'EPT_MCU_TEMP_DUP','Startbit', [ 0;],'SignalSize', [ 8;],'ByteOrder', 'LittleEndian','ValueType', 'UNSIGNED','Class', 'uint8','Signed', [ 0;],'Factor', [ 1;],'Offset', [ -40;],'Min', [ -40;],'Max', [ 210;],'Units', 'degC','Comment', '','StartBit', [ 8;]),struct('Name', 'EPT_MOTOR_TEMP_DUP','Startbit', [ 0;],'SignalSize', [ 8;],'ByteOrder', 'LittleEndian','ValueType', 'UNSIGNED','Class', 'uint8','Signed', [ 0;],'Factor', [ 1;],'Offset', [ -40;],'Min', [ -40;],'Max', [ 210;],'Units', 'degC','Comment', '','StartBit', [ 0;])}}
      settings: SourceProductName=Raptor
  raptor_data_read1 : Raptor_lib/Data Storage/raptor_data_read  dataName='EPT_MCU_FAULT_CAUSE'  dataShape=Scalar  idxSource=Input  idxRow=1  idxCol=1
      settings: SourceProductName=Raptor
  raptor_data_read2 : Raptor_lib/Data Storage/raptor_data_read  dataName='EPT_MCU_FAULT_LEVEL'  dataShape=Scalar  idxSource=Input  idxRow=1  idxCol=1
      settings: SourceProductName=Raptor
  raptor_data_read3 : Raptor_lib/Data Storage/raptor_data_read  dataName='EPT_MCU_FAULT_ID'  dataShape=Scalar  idxSource=Input  idxRow=1  idxCol=1
      settings: SourceProductName=Raptor
  raptor_data_read4 : Raptor_lib/Data Storage/raptor_data_read  dataName='Read_Motor_Temp'  dataShape=Scalar  idxSource=Input  idxRow=1  idxCol=1
      settings: SourceProductName=Raptor
  raptor_data_read5 : Raptor_lib/Data Storage/raptor_data_read  dataName='Read_Controller_Temp'  dataShape=Scalar  idxSource=Input  idxRow=1  idxCol=1
      settings: SourceProductName=Raptor
  wires:
  raptor_data_read4/1 -> raptor_can_txmsg/1  "EPT_MOTOR_TEMP_DUP"
  raptor_data_read5/1 -> raptor_can_txmsg/2  "EPT_MCU_TEMP_DUP"
  raptor_data_read1/1 -> raptor_can_txmsg/4  "EPT_MCU_FAULT_CAUSE"
  raptor_data_read3/1 -> raptor_can_txmsg/5  "EPT_MCU_FAULT_ID"
  raptor_data_read2/1 -> raptor_can_txmsg/3  "EPT_MCU_FAULT_LEVEL"

== system EPT/Foreground_TimeBase_5ms/CAN/CAN2_exec/Remote DA /Remote DA Status G21 (ESS-OBU#2) ==
  Trigger : TriggerPort  VariantControl=Variant  PortDimensions=1
  raptor_can_txmsg : Raptor_lib/CAN/raptor_can_txmsg  canDefinition=struct('dbcFile', 'EPTvsRemoteDA.dbc','message', 'Remote_DA_Status_G21','comment', '','signals', {{'EPT_BPOBU_CURR','EPT_BPOBU_FCCAP_DUP','EPT_BPOBU_RCAP','EPT_BPOBU_SOC_DUP','EPT_BPOBU_VOLT_DUP','EPT_HV_BUS_VOLT'}},'enabled', [ 1 1 1 1 1 1;],'canBus', '''CAN2''','messageID', [ 404877044;],'idMask', [ 536870911;],'payloadMask', [],'payloadValue', [],'period', [ 0;],'mailbox', '','queueSize', [ 1;],'label', [ 0;],'ver', [ 2;],'showID', [ 0;],'showRaw', [ 0;],'fill', [ 0;],'editID', [ 0;],'signalOrder', [ 1;])  canBus='CAN2'  queueSize=1  payloadMask=[]  payloadValue=[]  period=0  showID=0  label=0  idMask=hex2dec('1FFFFFFF')  fill=0  id=404877044  showRaw=0  signalOrder=1  signalInfo={{struct('Name', 'EPT_HV_BUS_VOLT','Startbit', [ 0;],'SignalSize', [ 8;],'ByteOrder', 'LittleEndian','ValueType', 'UNSIGNED','Class', 'uint8','Signed', [ 0;],'Factor', [ 0.4;],'Offset', [ 0;],'Min', [ 0;],'Max', [ 100;],'Units', '%(Max_Vbatt)','Comment', '','StartBit', [ 8;]),struct('Name', 'EPT_BPOBU_SOC_DUP','Startbit', [ 0;],'SignalSize', [ 8;],'ByteOrder', 'LittleEndian','ValueType', 'UNSIGNED','Class', 'uint8','Signed', [ 0;],'Factor', [ 0.5;],'Offset', [ -12.5;],'Min', [ -12.5;],'Max', [ 112.5;],'Units', '%','Comment', '','StartBit', [ 32;]),struct('Name', 'EPT_BPOBU_RCAP','Startbit', [ 0;],'SignalSize', [ 8;],'ByteOrder', 'LittleEndian','ValueType', 'UNSIGNED','Class', 'uint8','Signed', [ 0;],'Factor', [ 0.5;],'Offset', [ -12.5;],'Min', [ -12.5;],'Max', [ 112.5;],'Units', '%(Max Ah)','Comment', '','StartBit', [ 48;]),struct('Name', 'EPT_BPOBU_FCCAP_DUP','Startbit', [ 0;],'SignalSize', [ 8;],'ByteOrder', 'LittleEndian','ValueType', 'UNSIGNED','Class', 'uint8','Signed', [ 0;],'Factor', [ 0.4;],'Offset', [ 0;],'Min', [ 0;],'Max', [ 100;],'Units', '%(Max Ah)','Comment', '','StartBit', [ 40;]),struct('Name', 'EPT_BPOBU_CURR','Startbit', [ 0;],'SignalSize', [ 16;],'ByteOrder', 'LittleEndian','ValueType', 'UNSIGNED','Class', 'uint16','Signed', [ 0;],'Factor', [ 0.05;],'Offset', [ -800;],'Min', [ -800;],'Max', [ 800;],'Units', 'A','Comment', '','StartBit', [ 16;]),struct('Name', 'EPT_BPOBU_VOLT_DUP','Startbit', [ 0;],'SignalSize', [ 8;],'ByteOrder', 'LittleEndian','ValueType', 'UNSIGNED','Class', 'uint8','Signed', [ 0;],'Factor', [ 0.4;],'Offset', [ 0;],'Min', [ 0;],'Max', [ 100;],'Units', '%(Max_Vbatt)','Comment', '','StartBit', [ 0;])}}
      settings: SourceProductName=Raptor
  raptor_data_read : Raptor_lib/Data Storage/raptor_data_read  dataName='EPT_HV_BUS_VOLT'  dataShape=Scalar  idxSource=Input  idxRow=1  idxCol=1
      settings: SourceProductName=Raptor
  raptor_data_read1 : Raptor_lib/Data Storage/raptor_data_read  dataName='EPT_BPOBU_VOLT'  dataShape=Scalar  idxSource=Input  idxRow=1  idxCol=1
      settings: SourceProductName=Raptor
  raptor_data_read2 : Raptor_lib/Data Storage/raptor_data_read  dataName='EPT_BPOBU_SOC'  dataShape=Scalar  idxSource=Input  idxRow=1  idxCol=1
      settings: SourceProductName=Raptor
  raptor_data_read3 : Raptor_lib/Data Storage/raptor_data_read  dataName='EPT_BPOBU_RCAP'  dataShape=Scalar  idxSource=Input  idxRow=1  idxCol=1
      settings: SourceProductName=Raptor
  raptor_data_read4 : Raptor_lib/Data Storage/raptor_data_read  dataName='EPT_BPOBU_FCCAP'  dataShape=Scalar  idxSource=Input  idxRow=1  idxCol=1
      settings: SourceProductName=Raptor
  raptor_data_read5 : Raptor_lib/Data Storage/raptor_data_read  dataName='EPT_BPOBU_CURR'  dataShape=Scalar  idxSource=Input  idxRow=1  idxCol=1
      settings: SourceProductName=Raptor
  wires:
  raptor_data_read1/1 -> raptor_can_txmsg/5  "EPT_BPOBU_VOLT_DUP"
  raptor_data_read/1 -> raptor_can_txmsg/6  "EPT_HV_BUS_VOLT"
  raptor_data_read2/1 -> raptor_can_txmsg/4  "EPT_BPOBU_SOC_DUP"
  raptor_data_read3/1 -> raptor_can_txmsg/3  "EPT_BPOBU_RCAP"
  raptor_data_read4/1 -> raptor_can_txmsg/2  "EPT_BPOBU_FCCAP_DUP"
  raptor_data_read5/1 -> raptor_can_txmsg/1  "EPT_BPOBU_CURR"

== system EPT/Foreground_TimeBase_5ms/CAN/CAN2_exec/Remote DA /Remote DA Status G22 (ESS-OBU#3) ==
  Trigger : TriggerPort  VariantControl=Variant  PortDimensions=1
  Tcell Min/Max : Subsystem
  Vcell Min/Max : Subsystem
  raptor_can_txmsg : Raptor_lib/CAN/raptor_can_txmsg  canDefinition=struct('dbcFile', 'EPTvsRemoteDA.dbc','message', 'Remote_DA_Status_G22','comment', '','signals', {{'EPT_BPOBU_VCELL_MAX','EPT_BPOBU_TCELL_MAX','EPT_BPOBU_VCELL_MIN','EPT_BPOBU_TCELL_MIN','EPT_BPOBU_VCELL_MAX_NUM','EPT_BPOBU_VCELL_MIN_NUM','EPT_BPOBU_TCELL_MAX_NUM','EPT_BPOBU_TCELL_MIN_NUM'}},'enabled', [ 1 1 1 1 1 1 1 1;],'canBus', '''CAN2''','messageID', [ 404942580;],'idMask', [ 536870911;],'payloadMask', [],'payloadValue', [],'period', [ 0;],'mailbox', '','queueSize', [ 1;],'label', [ 0;],'ver', [ 2;],'showID', [ 0;],'showRaw', [ 0;],'fill', [ 0;],'editID', [ 0;],'signalOrder', [ 2;])  canBus='CAN2'  queueSize=1  payloadMask=[]  payloadValue=[]  period=0  showID=0  label=0  idMask=hex2dec('1FFFFFFF')  fill=0  id=404942580  showRaw=0  signalOrder=2  signalInfo={{struct('Name', 'EPT_BPOBU_VCELL_MIN_NUM','Startbit', [ 0;],'SignalSize', [ 8;],'ByteOrder', 'LittleEndian','ValueType', 'UNSIGNED','Class', 'uint8','Signed', [ 0;],'Factor', [ 1;],'Offset', [ 0;],'Min', [ 0;],'Max', [ 0;],'Units', '','Comment', '','StartBit', [ 40;]),struct('Name', 'EPT_BPOBU_VCELL_MIN','Startbit', [ 0;],'SignalSize', [ 8;],'ByteOrder', 'LittleEndian','ValueType', 'UNSIGNED','Class', 'uint8','Signed', [ 0;],'Factor', [ 0.01;],'Offset', [ 2;],'Min', [ 2;],'Max', [ 4.5;],'Units', 'V','Comment', '','StartBit', [ 16;]),struct('Name', 'EPT_BPOBU_VCELL_MAX_NUM','Startbit', [ 0;],'SignalSize', [ 8;],'ByteOrder', 'LittleEndian','ValueType', 'UNSIGNED','Class', 'uint8','Signed', [ 0;],'Factor', [ 1;],'Offset', [ 0;],'Min', [ 0;],'Max', [ 0;],'Units', '','Comment', '','StartBit', [ 32;]),struct('Name', 'EPT_BPOBU_VCELL_MAX','Startbit', [ 0;],'SignalSize', [ 8;],'ByteOrder', 'LittleEndian','ValueType', 'UNSIGNED','Class', 'uint8','Signed', [ 0;],'Factor', [ 0.01;],'Offset', [ 2;],'Min', [ 2;],'Max', [ 4.5;],'Units', 'V','Comment', '','StartBit', [ 0;]),struct('Name', 'EPT_BPOBU_TCELL_MIN_NUM','Startbit', [ 0;],'SignalSize', [ 8;],'ByteOrder', 'LittleEndian','ValueType', 'SIGNED','Class', 'int8','Signed', [ 1;],'Factor', [ 1;],'Offset', [ 0;],'Min', [ 0;],'Max', [ 0;],'Units', '','Comment', '','StartBit', [ 56;]),struct('Name', 'EPT_BPOBU_TCELL_MIN','Startbit', [ 0;],'SignalSize', [ 8;],'ByteOrder', 'LittleEndian','ValueType', 'UNSIGNED','Class', 'uint8','Signed', [ 0;],'Factor', [ 1;],'Offset', [ -40;],'Min', [ -40;],'Max', [ 210;],'Units', '','Comment', '','StartBit', [ 24;]),struct('Name', 'EPT_BPOBU_TCELL_MAX_NUM','Startbit', [ 0;],'SignalSize', [ 8;],'ByteOrder', 'LittleEndian','ValueType', 'UNSIGNED','Class', 'uint8','Signed', [ 0;],'Factor', [ 1;],'Offset', [ 0;],'Min', [ 0;],'Max', [ 0;],'Units', '','Comment', '','StartBit', [ 48;]),struct('Name', 'EPT_BPOBU_TCELL_MAX','Startbit', [ 0;],'SignalSize', [ 8;],'ByteOrder', 'LittleEndian','ValueType', 'UNSIGNED','Class', 'uint8','Signed', [ 0;],'Factor', [ 1;],'Offset', [ -40;],'Min', [ -40;],'Max', [ 210;],'Units', 'degC','Comment', '','StartBit', [ 8;])}}
      settings: SourceProductName=Raptor
  wires:
  Vcell Min/Max/3(Max Order) -> raptor_can_txmsg/5
  Vcell Min/Max/4(Min Order) -> raptor_can_txmsg/6
  Vcell Min/Max/2(Min) -> raptor_can_txmsg/3
  Vcell Min/Max/1(Max) -> raptor_can_txmsg/1
  Tcell Min/Max/3(Max Order) -> raptor_can_txmsg/7
  Tcell Min/Max/4(Min Order) -> raptor_can_txmsg/8
  Tcell Min/Max/2(Min) -> raptor_can_txmsg/4
  Tcell Min/Max/1(Max) -> raptor_can_txmsg/2
